simulink model "spg_hip"  (Simulink 8.1)
settings: Solver=ode4  StartTime=0  StopTime=24.2085  FixedStep=0.0005  MaxStep=0.01  RelTol=1e-3
values from neighbouring files (symbols this model uses):
  a = a+1    (= 2)    [final_process.m]    (also in runtrial.m = input('which side? R - 1, L - 2 '); simplot.m = [parameter(11) parameter(12); spgmodel.m = [parameter(11) parameter(12); spgsim.m = [parameter(11) parameter(12))
  b = b+1    (= 2)    [final_process.m]    (also in simplot.m = parameter(15:16); spgmodel.m = parameter(15:16); spgsim.m = parameter(15:16))
  r1 = 2.2952    [runtrial.m]    (also in simplot.m = parameter(9); spgmodel.m = parameter(9); spgsim.m = parameter(9))
  r2 = 0.0054    [runtrial.m]    (also in simplot.m = parameter(10); spgmodel.m = parameter(10); spgsim.m = parameter(10))
  s0 = data(1,2)    [simplot.m]    (also in spgmodel.m; spgsim.m)
  s1 = data(1,3)    [simplot.m]    (also in spgmodel.m; spgsim.m)
  Ta = parameter(13:14)    [simplot.m]    (also in spgmodel.m; spgsim.m)
  v0 = 0    [simplot.m]    (also in spgmodel.m; spgsim.m)
  W = parameter(1:2)    [simplot.m]    (also in spgmodel.m; spgsim.m)
  Wa = parameter(5:6)    [simplot.m]    (also in spgmodel.m; spgsim.m)
  Wv = parameter(3:4)    [simplot.m]    (also in spgmodel.m; spgsim.m)
  Wva = parameter(7:8)    [simplot.m]    (also in spgmodel.m; spgsim.m)
  x0 = data(1,4:end)    [simplot.m]    (also in spgmodel.m; spgsim.m)
settings Model: Creator=Arne  LastModifiedBy=chong
settings OptimizationCC: InitFltsAndDblsToZero=on
settings DebuggingCC: SaveWithParameterizedLinksMsg=none  SignalResolutionControl=TryResolveAllWithWarning  SolverPrmCheckMsg=none  MultiTaskDSMMsg=warning  MultiTaskCondExecSysMsg=none  StrictBusMsg=Warning
settings RTWCC: IncludeERTFirstTime=on
settings GRTTargetCC: TargetFcnLib=ansi_tfl_tmw.mat

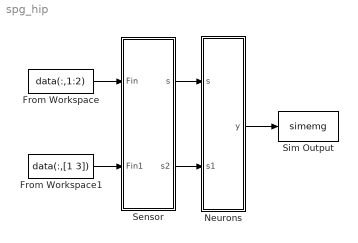
== system spg_hip ==
  From Workspace : FromWorkspace  VariableName=data(:,1:2)  SampleTime=0
  From Workspace1 : FromWorkspace  VariableName=data(:,[1 3])  SampleTime=0
  Neurons : Subsystem
  Sensor : Subsystem
  Sim Output : ToWorkspace  VariableName=simemg  SampleTime=-1
  wires:
  From Workspace/1 -> Sensor/1(Fin)
  Sensor/1(s) -> Neurons/1(s)
  Neurons/1(y) -> Sim Output/1
  Sensor/2(s2) -> Neurons/2(s1)
  From Workspace1/1 -> Sensor/2(Fin1)

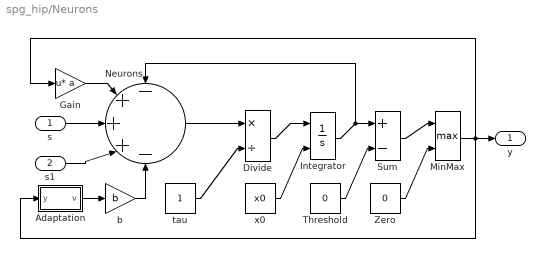
== system spg_hip/Neurons ==
  s : Inport
  s1 : Inport  Port=2
  Adaptation : Subsystem
  Divide : Product  Inputs=*/
  Gain : Gain  Gain=a  Multiplication=Matrix(u*K)
  Integrator : Integrator  InitialConditionSource=external
  MinMax : MinMax  Function=max  Inputs=2
  Neurons : Sum  Inputs=-+++-
  Sum : Sum  Inputs=+-
  Threshold : Constant  Value=0
  Zero : Constant  Value=0  VectorParams1D=off
  b : Gain  Gain=b
  tau : Constant  VectorParams1D=off
  x0 : Constant  Value=x0  VectorParams1D=off
  y : Outport
  wires:
  Integrator/1 -> Neurons/1, Sum/1
  Zero/1 -> MinMax/2
  MinMax/1 -> Adaptation/1(y), y/1, Gain/1
  Neurons/1 -> Divide/1
  tau/1 -> Divide/2
  Divide/1 -> Integrator/1
  x0/1 -> Integrator/2
  Adaptation/1(v) -> b/1
  Gain/1 -> Neurons/2
  Threshold/1 -> Sum/2
  Sum/1 -> MinMax/1
  s/1 -> Neurons/3
  b/1 -> Neurons/5
  s1/1 -> Neurons/4

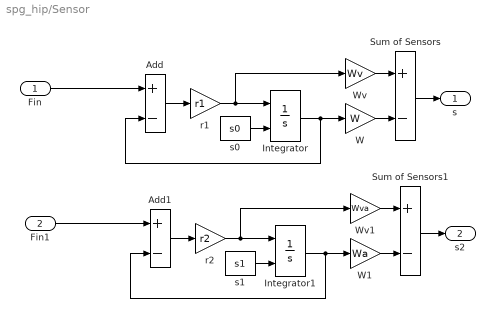
== system spg_hip/Sensor ==
  Fin : Inport
  Fin1 : Inport  Port=2
  Add : Sum  Inputs=+-
  Add1 : Sum  Inputs=+-
  Integrator : Integrator  InitialConditionSource=external
  Integrator1 : Integrator  InitialConditionSource=external
  Sum of Sensors : Sum  Inputs=+-
  Sum of Sensors1 : Sum  Inputs=+-
  W : Gain  Gain=W
  W1 : Gain  Gain=Wa
  Wv : Gain  Gain=Wv
  Wv1 : Gain  Gain=Wva
  r1 : Gain  Gain=r1
  r2 : Gain  Gain=r2
  s0 : Constant  Value=s0
  s1 : Constant  Value=s1
  s : Outport
  s2 : Outport  Port=2
  wires:
  Add/1 -> r1/1
  Integrator/1 -> Add/2, W/1
  r1/1 -> Integrator/1, Wv/1
  Fin/1 -> Add/1
  s0/1 -> Integrator/2
  Wv/1 -> Sum of Sensors/1
  W/1 -> Sum of Sensors/2
  Sum of Sensors/1 -> s/1
  Add1/1 -> r2/1
  Integrator1/1 -> Add1/2, W1/1
  r2/1 -> Integrator1/1, Wv1/1
  s1/1 -> Integrator1/2
  Wv1/1 -> Sum of Sensors1/1
  W1/1 -> Sum of Sensors1/2
  Sum of Sensors1/1 -> s2/1
  Fin1/1 -> Add1/1

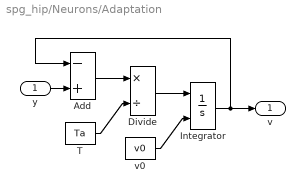
== system spg_hip/Neurons/Adaptation ==
  y : Inport
  Add : Sum  Inputs=-+
  Divide : Product  Inputs=*/
  Integrator : Integrator  InitialConditionSource=external
  T : Constant  Value=Ta  VectorParams1D=off
  v0 : Constant  Value=v0  VectorParams1D=off
  v : Outport
  wires:
  Integrator/1 -> Add/1, v/1
  y/1 -> Add/2
  T/1 -> Divide/2
  Add/1 -> Divide/1
  Divide/1 -> Integrator/1
  v0/1 -> Integrator/2
